simulink model "LCK"  (R2018b)
settings: Solver=FixedStepDiscrete  StartTime=0.0  StopTime=inf  FixedStep=0.01  RelTol=1e-3
PostLoadFcn:
  | if any(exist('dsrtsu_mdlpostloadfcn', 'file') ~= 0), dsrtsu_mdlpostloadfcn('Execute', bdroot); end
values from neighbouring files (symbols this model uses):
  C_DEG2RAD = 0.0175    [LCK_Macro.sldd]
  C_KPH2MPS = 0.2778    [LCK_Macro.sldd]
  C_NEARZERO = 0.0001    [LCK_Macro.sldd]
  C_ONE = 1.0    [LCK_Macro.sldd]
  C_RAD2DEG = 57.2958    [LCK_Macro.sldd]
  C_ZERO = 0.0    [LCK_Macro.sldd]
  k_accel_pedal_pos_per_speed_x : value not decoded    [LCK_LogicPara.sldd]
  k_accel_pedal_pos_per_speed_z : value not decoded    [LCK_LogicPara.sldd]
  k_brake_suprress_hold = 1000.0    [LCK_LogicPara.sldd]
  k_driver_appl_torque_filt = 50.0    [LCK_LogicPara.sldd]
  k_driver_suppression_hold_time = 3000.0    [LCK_LogicPara.sldd]
  k_hands_on_wheel_hold_msec = 500.0    [LCK_LogicPara.sldd]
  k_hands_on_wheel_torque_hi = 0.2    [LCK_LogicPara.sldd]
  k_hands_on_wheel_torque_lo = 0.15    [LCK_LogicPara.sldd]
  k_handsoff_delay_cycles = 50.0    [LCK_LogicPara.sldd]
  k_handsoff_torq_Lo_CR = 0.3    [LCK_LogicPara.sldd]
  k_handson_delay_cycles = 5.0    [LCK_LogicPara.sldd]
  k_HighAccel_suppress_hold = 3000.0    [LCK_LogicPara.sldd]
  k_HLR_suprress_hold = 3000.0    [LCK_LogicPara.sldd]
  k_hs_StrAng_CR_threshold_z : value not decoded    [LCK_LogicPara.sldd]
  k_LC_Exit_Switch = 0.0    [LCK_LogicPara.sldd]
  k_LCG_Configured = 1.0    [LCK_LogicPara.sldd]
  k_LCK_A0_Rdy2Act_UseConst = 0.0    [LCK_LogicPara.sldd]
  k_LCK_A0Fac_ActSta : value not decoded    [LCK_CtrlPara.sldd]
  k_LCK_A0Fac_DrvStm : value not decoded    [LCK_CtrlPara.sldd]
  k_LCK_A0Shift_LftCurv : value not decoded    [LCK_CtrlPara.sldd]
  k_LCK_A0Shift_RgtCurv : value not decoded    [LCK_CtrlPara.sldd]
  k_LCK_A0Shift_StraLan = 0.0    [LCK_CtrlPara.sldd]
  k_LCK_A0ShiftFac_Dy_LftCurv : value not decoded    [LCK_CtrlPara.sldd]
  k_LCK_A0ShiftFac_Dy_RgtCurv : value not decoded    [LCK_CtrlPara.sldd]
  k_LCK_A0ShiftFac_Vspd : value not decoded    [LCK_CtrlPara.sldd]
  k_LCK_accel_inhibit_thold = 35.0    [LCK_LogicPara.sldd]
  k_LCK_Active2Ready_Mask = 255.0    [LCK_LogicPara.sldd]
  k_LCK_CvatRateBks : value not decoded    [LCK_CtrlPara.sldd]
  k_LCK_CvatrBks : value not decoded    [LCK_CtrlPara.sldd]
  k_LCK_DFac_Dy : value not decoded    [LCK_CtrlPara.sldd]
  k_LCK_DFac_Dy_Curv : value not decoded    [LCK_CtrlPara.sldd]
  k_LCK_DFac_HaCurCen : value not decoded    [LCK_CtrlPara.sldd]
  k_LCK_DFac_HaCurSid : value not decoded    [LCK_CtrlPara.sldd]
  k_LCK_DFac_HadCurCen : value not decoded    [LCK_CtrlPara.sldd]
  k_LCK_DFac_HadCurSid : value not decoded    [LCK_CtrlPara.sldd]
  k_LCK_DFac_HadStrCen : value not decoded    [LCK_CtrlPara.sldd]
  k_LCK_DFac_HadStrSid : value not decoded    [LCK_CtrlPara.sldd]
  k_LCK_DFac_HaStrCen : value not decoded    [LCK_CtrlPara.sldd]
  k_LCK_DFac_HaStrSid : value not decoded    [LCK_CtrlPara.sldd]
  k_LCK_DFac_Rad : value not decoded    [LCK_CtrlPara.sldd]
  k_LCK_DFac_SA_CurCen : value not decoded    [LCK_CtrlPara.sldd]
  k_LCK_DFac_SA_CurSid : value not decoded    [LCK_CtrlPara.sldd]
  k_LCK_DFac_SA_StrCen : value not decoded    [LCK_CtrlPara.sldd]
  k_LCK_DFac_SA_StrSid : value not decoded    [LCK_CtrlPara.sldd]
  k_LCK_DFac_SS_CurCen : value not decoded    [LCK_CtrlPara.sldd]
  k_LCK_DFac_SS_CurSid : value not decoded    [LCK_CtrlPara.sldd]
  k_LCK_DFac_SS_StrCen : value not decoded    [LCK_CtrlPara.sldd]
  k_LCK_DFac_SS_StrSid : value not decoded    [LCK_CtrlPara.sldd]
  k_LCK_DFac_Vspd : value not decoded    [LCK_CtrlPara.sldd]
  k_LCK_DlyTm_DrvStim = 0.2    [LCK_CtrlPara.sldd]
  k_LCK_DTermMax = 2.0    [LCK_CtrlPara.sldd]
  k_LCK_DyBks_Curv : value not decoded    [LCK_CtrlPara.sldd]
  k_LCK_Enable_POOnly = 1.0    [LCK_LogicPara.sldd]
  k_LCK_Entry_DistBuffer = 0.1    [LCK_LogicPara.sldd]
  k_LCK_Fac_Vspd2RngThr_FalRec = 0.23    [LCK_CtrlPara.sldd]
  k_LCK_Ffw_CvatSwh = 0.0    [LCK_CtrlPara.sldd]
  k_LCK_Ffw_DyBks : value not decoded    [LCK_CtrlPara.sldd]
  k_LCK_Ffw_TimCon_CmdFlt = 0.0    [LCK_CtrlPara.sldd]
  k_LCK_FfwDeltaFac_Rad_Lft : value not decoded    [LCK_CtrlPara.sldd]
  k_LCK_FfwDeltaFac_Rad_Rgt : value not decoded    [LCK_CtrlPara.sldd]
  k_LCK_FfwDeltaFac_Vspd : value not decoded    [LCK_CtrlPara.sldd]
  k_LCK_FfwFac_CvatRate_Lft : value not decoded    [LCK_CtrlPara.sldd]
  k_LCK_FfwFac_CvatRate_Rgt : value not decoded    [LCK_CtrlPara.sldd]
  k_LCK_FfwFac_Dy : value not decoded    [LCK_CtrlPara.sldd]
  k_LCK_FfwFac_Rad_Lft : value not decoded    [LCK_CtrlPara.sldd]
  k_LCK_FfwFac_Rad_Rgt : value not decoded    [LCK_CtrlPara.sldd]
  k_LCK_FfwFac_Vspd : value not decoded    [LCK_CtrlPara.sldd]
  k_LCK_FfwTorq_Cvat : value not decoded    [LCK_CtrlPara.sldd]
  k_LCK_HAFac_ActSta : value not decoded    [LCK_CtrlPara.sldd]
  k_LCK_HAFac_DrvStm : value not decoded    [LCK_CtrlPara.sldd]
  k_LCK_HaloTime = 2000.0    [LCK_LogicPara.sldd]
  k_LCK_HaloTime_Switch = 0.0    [LCK_LogicPara.sldd]
  k_LCK_HARFac_ActSta : value not decoded    [LCK_CtrlPara.sldd]
  k_LCK_HARFac_DrvStm : value not decoded    [LCK_CtrlPara.sldd]
  k_LCK_Hed_DyBks : value not decoded    [LCK_CtrlPara.sldd]
  k_LCK_HedAngDiffX : value not decoded    [LCK_CtrlPara.sldd]
  k_LCK_HedAngRateDiffX : value not decoded    [LCK_CtrlPara.sldd]
  k_LCK_HndsOnWhel_DlyTm_Idl2Rdy = 0.0    [LCK_LogicPara.sldd]
  k_LCK_host_veh_width = 1.86    [LCK_LogicPara.sldd]
  k_LCK_Idle2Ready_Mask = 239.0    [LCK_LogicPara.sldd]
  k_LCK_Junc_SusTime = 1.0    [LCK_LogicPara.sldd]
  k_LCK_KpKdDecSlopeLmt = 10.0    [LCK_CtrlPara.sldd]
  k_LCK_KpKdIncSlopeLmt = 5.0    [LCK_CtrlPara.sldd]
  k_LCK_Lat_Ctrl_DFac_Lft = 1.0    [LCK_CtrlPara.sldd]
  k_LCK_Lat_Ctrl_DFac_Rgt = 1.05    [LCK_CtrlPara.sldd]
  k_LCK_Lat_Ctrl_Kd = 0.8    [LCK_CtrlPara.sldd]
  k_LCK_Lat_Ctrl_Ki = 0.5    [LCK_CtrlPara.sldd]
  k_LCK_Lat_Ctrl_Kp = 0.7    [LCK_CtrlPara.sldd]
  k_LCK_Lat_Ctrl_Kp_NearGain = 0.7    [LCK_CtrlPara.sldd]
  k_LCK_Lat_Ctrl_PFac_Lft = 1.0    [LCK_CtrlPara.sldd]
  k_LCK_Lat_Ctrl_PFac_Rgt = 1.05    [LCK_CtrlPara.sldd]
  k_LCK_Lat_Ctrl_TimCon_CmdFlt = 5.0    [LCK_CtrlPara.sldd]
  k_LCK_Lat_DFac_Rad : value not decoded    [LCK_CtrlPara.sldd]
  k_LCK_Lat_DFac_SS_Cur : value not decoded    [LCK_CtrlPara.sldd]
  k_LCK_Lat_DFac_SS_Str : value not decoded    [LCK_CtrlPara.sldd]
  k_LCK_Lat_DFac_Vspd : value not decoded    [LCK_CtrlPara.sldd]
  k_LCK_Lat_DyBks : value not decoded    [LCK_CtrlPara.sldd]
  k_LCK_Lat_IFac_Rad : value not decoded    [LCK_CtrlPara.sldd]
  k_LCK_Lat_IFac_Vspd : value not decoded    [LCK_CtrlPara.sldd]
  k_LCK_Lat_ILmtFac_Dy_CurvLan : value not decoded    [LCK_CtrlPara.sldd]
  k_LCK_Lat_ILmtFac_Dy_StraLan : value not decoded    [LCK_CtrlPara.sldd]
  k_LCK_Lat_ILmtFac_Rad : value not decoded    [LCK_CtrlPara.sldd]
  k_LCK_Lat_ILmtFac_Rad_NearGain = 1.0    [LCK_CtrlPara.sldd]
  k_LCK_Lat_ILmtFac_Vspd_CurvLan : value not decoded    [LCK_CtrlPara.sldd]
  k_LCK_Lat_ILmtFac_Vspd_StraLan : value not decoded    [LCK_CtrlPara.sldd]
  k_LCK_Lat_ITermLmt_Dy = 1.0    [LCK_CtrlPara.sldd]
  k_LCK_Lat_KpKdDecSlopeLmt = 10.0    [LCK_CtrlPara.sldd]
  k_LCK_Lat_KpKdIncSlopeLmt = 10.0    [LCK_CtrlPara.sldd]
  k_LCK_Lat_PFac_Dy_InnLftCur : value not decoded    [LCK_CtrlPara.sldd]
  k_LCK_Lat_PFac_Dy_InnRgtCur : value not decoded    [LCK_CtrlPara.sldd]
  k_LCK_Lat_PFac_Dy_OutLftCur : value not decoded    [LCK_CtrlPara.sldd]
  k_LCK_Lat_PFac_Dy_OutRgtCur : value not decoded    [LCK_CtrlPara.sldd]
  k_LCK_Lat_PFac_Dy_Str : value not decoded    [LCK_CtrlPara.sldd]
  k_LCK_Lat_PFac_Rad : value not decoded    [LCK_CtrlPara.sldd]
  ... (+153 more)
undefined symbols (not defined in the file or in its folder): k_LCK_CurvBks, K_LCK_SPA0A1A2_LMRngCmp_y
libraries: LateralControl_fcns_lib x59, simulink x24
(part 35 of 47)

== system LCK/Lateral_Control_Module/LCK_State_Ctrl/LCK_Mode_Transition/SP_conf_Judgement ==
  note: 0x0: Invalid
      | 0x1: Low
      | 0x2: Med
      | 0x3: MedHigh
      | 0x4: High
  veh_speed_kph : Inport
  SP_conf : Inport  Port=2
  Junction : Inport  Port=3
  Constant50 : Constant  Tag={'output',{'type','Int32'},'date',737237.63746362273}  Description=_GWMAB30P3.LCK.000_46_  Value=0
  Constant51 : Constant  Tag={'output',{'type','Int32'},'date',737237.63746376161}  Description=_GWMAB30P3.LCK.000_47_
  Constant52 : Constant  Tag={'output',{'type','Int32'},'date',737237.63746390049}  Description=_GWMAB30P3.LCK.000_48_  Value=2
  Data Type Conversion16 : DataTypeConversion  Description=_GWMAB30P4.LCK.000_127_
  Data Type Conversion25 : DataTypeConversion  Description=_GWMAB30P4.LCK.000_136_
  Data Type Conversion26 : DataTypeConversion  Description=_GWMAB30P4.LCK.000_137_
  Delay_Trig : LateralControl_fcns_lib/Delay_Trig  SystemSampleTime=-1
  Delay_Trig1 : LateralControl_fcns_lib/Delay_Trig  SystemSampleTime=-1
  Delay_Trig2 : LateralControl_fcns_lib/Delay_Trig  SystemSampleTime=-1
  Logical Operator9 : Logic  Tag={'date',737237.63747025467}  Description=_GWMAB30P3.LCK.000_84_  Operator=OR  Inputs=3  AllPortsSameDT=off  OutDataTypeStr=boolean
  Relational Operator44 : RelationalOperator  Tag={'date',737237.6374723264}  Description=_GWMAB30P3.LCK.000_94_  Operator===  OutDataTypeStr=boolean  RndMeth=Nearest
  Relational Operator45 : RelationalOperator  Tag={'date',737237.63747245376}  Description=_GWMAB30P3.LCK.000_95_  Operator===  OutDataTypeStr=boolean  RndMeth=Nearest
  Relational Operator8 : RelationalOperator  Tag={'date',737237.63747402781}  Description=_GWMAB30P3.LCK.000_104_  Operator===  OutDataTypeStr=boolean  RndMeth=Nearest
  Switch63 : Switch  Tag={'output',{'type','Float32'},'threshold',{'type','Int32'},'date',737531.80846928246}  Description=_GACA26P4.LCK.000_43_  Criteria=u2 > Threshold  Threshold=0.5
  Switch64 : Switch  Tag={'output',{'type','Float32'},'threshold',{'type','Int32'},'date',737531.80875576392}  Description=_GACA26P4.LCK.000_44_  Criteria=u2 > Threshold  Threshold=0.5
  Switch68 : Switch  Tag={'output',{'type','Float32'},'threshold',{'type','Int32'},'date',737531.80856611114}  Description=_GACA26P4.LCK.000_48_  Criteria=u2 > Threshold  Threshold=0.5
  Switch70 : Switch  Tag={'output',{'type','Float32'},'threshold',{'type','Int32'},'date',737531.80889267358}  Description=_GACA26P4.LCK.000_50_  Criteria=u2 > Threshold  Threshold=0.5
  Use_Constant_SPP_Timer : Constant  Tag={'output',{'name','$P','class','EXTERN_CAL','type','Bool'},'date',737531.63716577541}  Description=_GACA26P4.LCK.000_57_  Value=k_Use_Constant_SPP_Timer
  k_LCK_SP_Conf_Low_JuncTm : Constant  Tag={'output',{'name','$P','class','EXTERN_CAL','type','Float32'},'date',737531.64170672453}  Description=_GACA26P4.LCK.000_67_  Value=k_LCK_SP_Conf_Low_JuncTm
  k_LCK_SP_Conf_Med_JuncTm : Constant  Tag={'output',{'name','$P','class','EXTERN_CAL','type','Float32'},'date',737531.63831533561}  Description=_GACA26P4.LCK.000_68_  Value=k_LCK_SP_Conf_Med_JuncTm
  k_LCK_SPconfInvld_DlyTm_Rdy2Idl : Constant  Tag={'output',{'name','$P','class','EXTERN_CAL','type','Float32'},'date',737246.86453196756}  Description=_GWMAB30P3.LCK.000_143_  Value=k_LCK_SPconfInvld_DlyTm_Rdy2Idl
  k_LCK_SPconfLow_DlyTm_Rdy2Idl : Constant  Tag={'output',{'name','$P','class','EXTERN_CAL','type','Float32'},'date',737531.64128429396}  Description=_GWMAB30P3.LCK.000_144_  Value=k_LCK_SPconfLow_DlyTm_Rdy2Idl
  k_LCK_SPconfLow_DlyTm_Rdy2Idl_Table : Lookup_n-D  Tag={'input',{'name','$P','class','EXTERN_CAL','type','Float32'},'output',{'type','Float32'},'table',{'name','$P','class','EXTERN_CAL','type','Float32'},'date',737531.7879730555}  Description=_GACA26P4.LCK.000_69_  NumberOfTableDimensions=1  BreakpointsForDimension1=k_LCK_SPconfLow_DlyTm_Rdy2Idl_x  Table=k_LCK_SPconfLow_DlyTm_Rdy2Idl_z  ExtrapMethod=Clip  InternalRulePriority=Speed  RndMeth=Simplest  InputSameDT=on
  k_LCK_SPconfMed_DlyTm_Rdy2Idl : Constant  Tag={'output',{'name','$P','class','EXTERN_CAL','type','Float32'},'date',737531.64166221069}  Description=_GWMAB30P3.LCK.000_145_  Value=k_LCK_SPconfMed_DlyTm_Rdy2Idl
  k_LCK_SPconfMed_DlyTm_Rdy2Idl_Table : Lookup_n-D  Tag={'input',{'name','$P','class','EXTERN_CAL','type','Float32'},'output',{'type','Float32'},'table',{'name','$P','class','EXTERN_CAL','type','Float32'},'date',737531.78800032404}  Description=_GACA26P4.LCK.000_70_  NumberOfTableDimensions=1  BreakpointsForDimension1=k_LCK_SPconfMed_DlyTm_Rdy2Idl_x  Table=k_LCK_SPconfMed_DlyTm_Rdy2Idl_z  ExtrapMethod=Clip  InternalRulePriority=Speed  RndMeth=Simplest  InputSameDT=on
  SP_conf_Judgement : Outport
  wires:
  Delay_Trig1/1 -> Logical Operator9/2
  Data Type Conversion16/1 -> Delay_Trig/1
  k_LCK_SP_Conf_Med_JuncTm/1 -> Switch70/1
  Constant52/1 -> Relational Operator45/2
  Relational Operator45/1 -> Data Type Conversion26/1
  Relational Operator44/1 -> Data Type Conversion25/1
  [SP_conf] -> Relational Operator44/1
  Constant51/1 -> Relational Operator44/2
  k_LCK_SPconfInvld_DlyTm_Rdy2Idl/1 -> Delay_Trig/2
  Relational Operator8/1 -> Data Type Conversion16/1
  k_LCK_SPconfLow_DlyTm_Rdy2Idl/1 -> Switch63/1
  [SP_conf] -> Relational Operator45/1
  Data Type Conversion25/1 -> Delay_Trig1/1
  Delay_Trig2/1 -> Logical Operator9/3
  Switch64/1 -> Delay_Trig2/2
  Data Type Conversion26/1 -> Delay_Trig2/1
  veh_speed_kph/1 -> k_LCK_SPconfLow_DlyTm_Rdy2Idl_Table/1, k_LCK_SPconfMed_DlyTm_Rdy2Idl_Table/1
  Constant50/1 -> Relational Operator8/2
  Junction/1 -> [Junction], Switch68/2
  Use_Constant_SPP_Timer/1 -> Switch63/2, Switch64/2
  Switch63/1 -> Delay_Trig1/2
  Delay_Trig/1 -> Logical Operator9/1
  k_LCK_SPconfLow_DlyTm_Rdy2Idl_Table/1 -> Switch68/3
  Switch68/1 -> Switch63/3
  Switch70/1 -> Switch64/3
  k_LCK_SPconfMed_DlyTm_Rdy2Idl_Table/1 -> Switch70/3
  k_LCK_SPconfMed_DlyTm_Rdy2Idl/1 -> Switch64/1
  [Junction] -> Switch70/2
  k_LCK_SP_Conf_Low_JuncTm/1 -> Switch68/1
  SP_conf/1 -> [SP_conf], Relational Operator8/1
  Logical Operator9/1 -> SP_conf_Judgement/1
